simulink library "NelinSys"  (Simulink 2.20)
values from neighbouring files (symbols this model uses):
  v = menu('EXACT LINEARIZATION (demo simulations)',    'Exact linearization of SISO system',    'Exact linearization of MIMO system',    'System with unstable zero dynamics')    [demos_exakt.m]    (also in demos_fp.m = menu('PHASE PLANE ANALYSIS (demo simulations)',    '2nd-Orde; demos_gs.m = menu('GAIN SCHEDULING (demo simulations)',    'Input and out)
  x1 = x(j)    [fazrov_auton2.m]
  x2 = x(j+1)    [fazrov_auton2.m]    (also in fazrov_typ1.m = get_param(get_param(gcbh,'Parent'),'UserData'))
undefined symbols (not defined in the file or in its folder): sfunvxy
libraries: simulink x5
(part 2 of 2)

== system NelinSys/Nonlinear Systems Synthesis/Gain Scheduling Blocks ==
  note: w(t)
  note: x(t)
  note: u(t)
  Controller synthesis for SISO systems : Subsystem
      settings: OpenFcn=progzos
      mask Type: Gain Scheduling - controller design for SISO systems
      mask Display: disp('GS SISO');
  Demonstracne simulacie : Subsystem
      settings: OpenFcn=demos_gs
      mask Type: Gain Scheduling - demo simulations
      mask Display: disp('Demo simulations');
  State-space gain-scheduling controller for SISO systems : Subsystem  mask(State-space gain-scheduling controller for SISO systems){n=2, vzorec=-(-w^(1/2)+4*w)/w*x1+4*w+1/2*(-w^(1/2)+8*w-16*w^(3/2))/w*(x2-w), vzorecP=0}
      mask prompts: n "System order (number of states):"; vzorec "Control action - symbolic expression:"; vzorecP "Control action - variable identifier:"
      mask help:
      | Block carries out control action of a state-space controller for nonlinear SISO system. The control action equation u = u(w,x) can be specified either as a symbolic expression or as an identifier of a symbolic variable.
      |
      | Block is typically used in place of a state-space controller designed via gain scheduling - to design such controller, "ProgZos.m" application can be used - however, in fact, the block can perform arbitrary control action specified by equation u = u(w,x), where w(t) is desired value and x(t) is states vector.
      |
      | For a detailed description of block parameters, click "Help" button below.
      mask init:
      | % Overenie spravnosti zadania parametrov bloku %
      | if isempty(n)
      |    error(['System order not specified - cannot continue!']);
      | end
      | 
      | if ~isempty(vzorec) & (vzorecP == 0)
      |    vzorec = sym(vzorec);
      | elseif isempty(vzorec) & (any(vzorecP ~= 0))
      |    vzorec = sym(vzorecP);
      | else
      |    error(['Equation for control action not specified or specified more than once - cannot continue!']);
      | end
      | 
      | % Zisti si symbolicke premenne, ktore vystupuju vo vyraze %
      | prem = strrep(strrep(findsym(sym(vzorec)),', ',''),',',' ');
      | 
      | % Premenne x1, x2, ..., xN su korektne, preskoc ich %
      | for k = 1 : n
      |    prem = strrep(prem, sprintf('x%d',k), '');
      | end
      | 
      | % Aj "w" je korektne, preskoc aj to %
      | prem = strrep(prem,'w','');
      | 
      | % Ak niektory retazec nezostal prazdny, vyhlas chybu %
      | if ~isempty(prem)
      |    error(['Unknown symbol in control action equation - cannot continue!']);
      | end
      | 
      | % Nahradenie identifikatorov "xI" identifikatormi "u(I+1)" a "w" pomocou "u(1)" %
      | co_str = '{''w'',''x1'; cim_str = '{''u(1)'',''u(2)';
      | 
      | for k = 2 : n
      |     co_str = sprintf('%s'',''x%d', co_str, k);
      |     cim_str = sprintf('%s'',''u(%d)', cim_str, k+1);
      | end
      | 
      | co_str = strcat(co_str, '''}'); cim_str = strcat(cim_str, '''}');
      | vzorec = eval(sprintf('subs(vzorec,%s,%s)', co_str, cim_str));
      mask Help: web(fullfile(cd,'help','gs_siso.html'));
      mask Display: disp('GS SISO\nu = u(w,x)');

== system NelinSys/Nonlinear Systems Synthesis/Nonlinear MIMO system (State-Space model) ==
  Vstup : Inport  Port=1  PortWidth=-1  SampleTime=-1
  Demux : Demux  Outputs=[nout n]
  S-funkcia realizujuca nelinearny system : S-Function  FunctionName=stavp_mimo  Parameters=n,nin,nout,F,G,H,pp  PortCounts=[]  SFunctionModules=''
  Vystup : Outport  Port=1  InitialOutput=0
  Stavovy vektor : Outport  Port=2
  wires:
  Demux/2 -> Stavovy vektor/1
  Demux/1 -> Vystup/1
  S-funkcia realizujuca nelinearny system/1 -> Demux/1
  Vstup/1 -> S-funkcia realizujuca nelinearny system/1

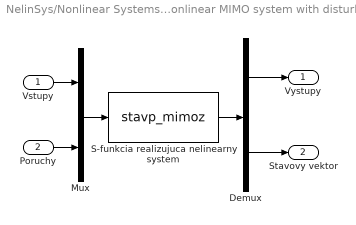
== system NelinSys/Nonlinear Systems Synthesis/Nonlinear MIMO system with disturbance ==
  Vstupy : Inport  Port=1  PortWidth=-1  SampleTime=-1
  Poruchy : Inport  Port=2  PortWidth=-1  SampleTime=-1
  Demux : Demux  Outputs=[nout n]
  Mux : Mux  Inputs=2
  S-funkcia realizujuca nelinearny system : S-Function  FunctionName=stavp_mimoz  Parameters=n,nin,nout,nz,F,G,H,E,pp  PortCounts=[]  SFunctionModules=''
  Vystupy : Outport  Port=1  InitialOutput=0
  Stavovy vektor : Outport  Port=2
  wires:
  S-funkcia realizujuca nelinearny system/1 -> Demux/1
  Demux/1 -> Vystupy/1
  Demux/2 -> Stavovy vektor/1
  Mux/1 -> S-funkcia realizujuca nelinearny system/1
  Vstupy/1 -> Mux/1
  Poruchy/1 -> Mux/2

== system NelinSys/Nonlinear Systems Synthesis/Nonlinear SISO system (State-Space model) ==
  Vstup : Inport  Port=1  PortWidth=-1  SampleTime=-1
  Demux : Demux  Outputs=[1 n]
  S-funkcia realizujuca nelinearny system : S-Function  FunctionName=stavp_siso  Parameters=n,F,G,H,pp  PortCounts=[]  SFunctionModules=''
  Vystup : Outport  Port=1  InitialOutput=0
  Stavovy vektor : Outport  Port=2
  wires:
  Vstup/1 -> S-funkcia realizujuca nelinearny system/1
  S-funkcia realizujuca nelinearny system/1 -> Demux/1
  Demux/1 -> Vystup/1
  Demux/2 -> Stavovy vektor/1

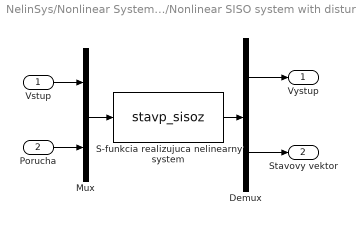
== system NelinSys/Nonlinear Systems Synthesis/Nonlinear SISO system with disturbance ==
  Vstup : Inport  Port=1  PortWidth=-1  SampleTime=-1
  Porucha : Inport  Port=2  PortWidth=-1  SampleTime=-1
  Demux : Demux  Outputs=[1 n]
  Mux : Mux  Inputs=2
  S-funkcia realizujuca nelinearny system : S-Function  FunctionName=stavp_sisoz  Parameters=n,F,G,H,E,pp  PortCounts=[]  SFunctionModules=''
  Vystup : Outport  Port=1  InitialOutput=0
  Stavovy vektor : Outport  Port=2
  wires:
  Demux/2 -> Stavovy vektor/1
  Demux/1 -> Vystup/1
  S-funkcia realizujuca nelinearny system/1 -> Demux/1
  Mux/1 -> S-funkcia realizujuca nelinearny system/1
  Vstup/1 -> Mux/1
  Porucha/1 -> Mux/2

== system NelinSys/Nonlinear Systems Synthesis/Exact Linearization Blocks/Controller synthesis for MIMO systems ==

== system NelinSys/Nonlinear Systems Synthesis/Exact Linearization Blocks/Controller synthesis for SISO systems ==

== system NelinSys/Nonlinear Systems Synthesis/Exact Linearization Blocks/Coordinates transformation for MIMO systems ==
  x : Inport  Port=1  PortWidth=-1  SampleTime=-1
  S-funkcia realizujuca transformaciu suradnic : S-Function  FunctionName=transf_mimo  Parameters=n,r,Z  PortCounts=[]  SFunctionModules=''
  q : Outport  Port=1
  wires:
  x/1 -> S-funkcia realizujuca transformaciu suradnic/1
  S-funkcia realizujuca transformaciu suradnic/1 -> q/1

== system NelinSys/Nonlinear Systems Synthesis/Exact Linearization Blocks/Coordinates transformation for SISO systems ==
  x : Inport  Port=1  PortWidth=-1  SampleTime=-1
  S-funkcia realizujuca transformaciu suradnic : S-Function  FunctionName=transf_surad  Parameters=n,r,Z  PortCounts=[]  SFunctionModules=''
  q : Outport  Port=1
  wires:
  x/1 -> S-funkcia realizujuca transformaciu suradnic/1
  S-funkcia realizujuca transformaciu suradnic/1 -> q/1

== system NelinSys/Nonlinear Systems Synthesis/Exact Linearization Blocks/Demonstracne simulacie ==

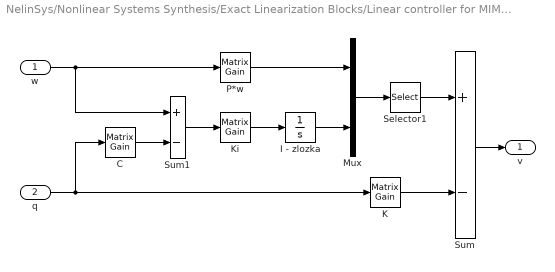
== system NelinSys/Nonlinear Systems Synthesis/Exact Linearization Blocks/Linear controller for MIMO systems ==
  w : Inport  Port=1  PortWidth=-1  SampleTime=-1
  q : Inport  Port=2  PortWidth=-1  SampleTime=-1
  C : simulink/Linear/Matrix Gain  K=C
  I - zlozka : Integrator  ExternalReset=none  InitialConditionSource=internal  InitialCondition=0  LimitOutput=off  UpperSaturationLimit=inf  LowerSaturationLimit=-inf  ShowSaturationPort=off  ShowStatePort=off  AbsoluteTolerance=auto
  K : simulink/Linear/Matrix Gain  K=K
  Ki : simulink/Linear/Matrix Gain  K=Ki
  Mux : Mux  Inputs=2
  P*w : simulink/Linear/Matrix Gain  K=P
  Selector1 : Selector  Elements=~integ*(1:nout)+integ*(nout+1:2*nout)  InputPortWidth=2*nout
  Sum : Sum  Inputs=+-
  Sum1 : Sum  Inputs=+-
  v : Outport  Port=1  InitialOutput=0
  wires:
  Sum/1 -> v/1
  K/1 -> Sum/2
  Ki/1 -> I - zlozka/1
  C/1 -> Sum1/2
  Sum1/1 -> Ki/1
  Selector1/1 -> Sum/1
  Mux/1 -> Selector1/1
  I - zlozka/1 -> Mux/2
  q/1 -> K/1, C/1
  P*w/1 -> Mux/1
  w/1 -> Sum1/1, P*w/1

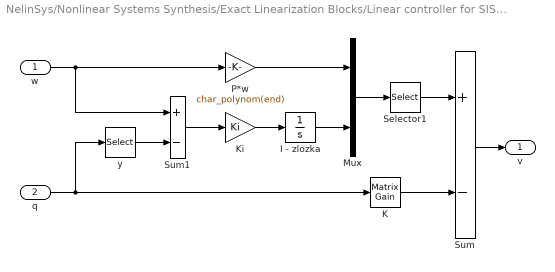
== system NelinSys/Nonlinear Systems Synthesis/Exact Linearization Blocks/Linear controller for SISO systems ==
  w : Inport  Port=1  PortWidth=-1  SampleTime=-1
  q : Inport  Port=2  PortWidth=-1  SampleTime=-1
  I - zlozka : Integrator  ExternalReset=none  InitialConditionSource=internal  InitialCondition=0  LimitOutput=off  UpperSaturationLimit=inf  LowerSaturationLimit=-inf  ShowSaturationPort=off  ShowStatePort=off  AbsoluteTolerance=auto
  K : simulink/Linear/Matrix Gain  K=K
  Ki : Gain  Gain=Ki
  Mux : Mux  Inputs=2
  P*w : Gain  Gain=char_polynom(end)
  Selector1 : Selector  Elements=integ+1  InputPortWidth=2
  Sum : Sum  Inputs=+-
  Sum1 : Sum  Inputs=+-
  y : Selector  Elements=1  InputPortWidth=r
  v : Outport  Port=1  InitialOutput=0
  wires:
  w/1 -> P*w/1, Sum1/1
  P*w/1 -> Mux/1
  q/1 -> y/1, K/1
  I - zlozka/1 -> Mux/2
  Mux/1 -> Selector1/1
  Selector1/1 -> Sum/1
  Sum1/1 -> Ki/1
  y/1 -> Sum1/2
  Ki/1 -> I - zlozka/1
  K/1 -> Sum/2
  Sum/1 -> v/1

== system NelinSys/Nonlinear Systems Synthesis/Exact Linearization Blocks/Linearizing control law for MIMO systems ==
  v : Inport  Port=1  PortWidth=-1  SampleTime=-1
  x : Inport  Port=2  PortWidth=-1  SampleTime=-1
  Mux : Mux  Inputs=2
  "s-funkcia pocita akcny zasah na zaklade x,v " : S-Function  FunctionName=lineariz_mimo  Parameters=n,nout,vzorec  PortCounts=[]  SFunctionModules=''
  u : Outport  Port=1  InitialOutput=0
  wires:
  "s-funkcia pocita akcny zasah na zaklade x,v "/1 -> u/1
  Mux/1 -> "s-funkcia pocita akcny zasah na zaklade x,v "/1
  v/1 -> Mux/1
  x/1 -> Mux/2

== system NelinSys/Nonlinear Systems Synthesis/Exact Linearization Blocks/Linearizing control law for SISO systems ==
  v : Inport  Port=1  PortWidth=-1  SampleTime=-1
  x : Inport  Port=2  PortWidth=-1  SampleTime=-1
  Mux : Mux  Inputs=2
  "s-funkcia pocita akcny zasah na zaklade x,v " : S-Function  FunctionName=lineariz_vztah  Parameters=n,vzorec  PortCounts=[]  SFunctionModules=''
  u : Outport  Port=1  InitialOutput=0
  wires:
  "s-funkcia pocita akcny zasah na zaklade x,v "/1 -> u/1
  Mux/1 -> "s-funkcia pocita akcny zasah na zaklade x,v "/1
  v/1 -> Mux/1
  x/1 -> Mux/2

== system NelinSys/Nonlinear Systems Synthesis/Gain Scheduling Blocks/Controller synthesis for SISO systems ==

== system NelinSys/Nonlinear Systems Synthesis/Gain Scheduling Blocks/Demonstracne simulacie ==

== system NelinSys/Nonlinear Systems Synthesis/Gain Scheduling Blocks/State-space gain-scheduling controller for SISO systems ==
  w : Inport  Port=1  PortWidth=-1  SampleTime=-1
  x : Inport  Port=2  PortWidth=-1  SampleTime=-1
  Mux : Mux  Inputs=2
  s-funkcia realizujuca regulator : S-Function  FunctionName=gs_siso  Parameters=n,vzorec  PortCounts=[]  SFunctionModules=''
  u : Outport  Port=1  InitialOutput=0
  wires:
  Mux/1 -> s-funkcia realizujuca regulator/1
  x/1 -> Mux/2
  s-funkcia realizujuca regulator/1 -> u/1
  w/1 -> Mux/1
